simulink library "ITKLib"  (R2022b)
settings: Solver=FixedStepDiscrete  StartTime=0.0  StopTime=10.0  FixedStep=0.01  RelTol=1e-3  EnableMultiTasking=on
values from neighbouring files (symbols this model uses):
  Glb_WhlRollgRd_SC = single(0.36)    [init_Global.m]
undefined symbols (not defined in the file or in its folder): docblock, SlDemoSign, SlDemoSign_Positive_SC, TaskTime_100ms_SC, TaskTime_10ms_SC, VehRefSpd_vMaxRefSpd_C
libraries: simulink x51, $bdroot x45, ITKLib_V14 x1
(part 4 of 10)

== system ITKLib/BasicOperators/AtanDeg ==
  u : Inport
  1-D Lookup Table3 : Lookup_n-D  NumberOfTableDimensions=1  BreakpointsForDimension1=[0,0.00153414561609111,0.00306829845373796,0.00460246573463227,0.00613665468073772,0.00767087251442592,0.00920512645861245,0.0107394237368928,0.0122737715736787,0.0138081771943337,0.0153426478253099,0.0168771906942835,0.0184118130302918,0.0199465220638685,0.0214813250271809,0.0230162291541658,0.0245512416806661,0.0260863698445676,0.0276216208859351,0.0291570020471495,0.0306925205730446,0.0322281837110438,0.0337639987112974,0.0352999728268193,0.0368361133136247,0.0383724274308672,0.0399089224409762,0.0414456056097949,0.0429824842067175,0.0445195655048274,0.0460568567810355,0.0475943653162178,0.0491320983953542,0.0506700633076669,0.0522082673467589,0.0537467178107533,0.0552854220024318,0.0568243872293744,0.0583636208040985,0.0599031300441989,0.0614429222724871,0.0629830048171318,0.0645233850117991,0.0660640701957925,0.0676050677141943,0.0691463849180061,0.0706880291642902,0.0722300078163106,0.0737723282436753,0.0753149978224779,0.0768580239354395,0.0784014139720518,0.0799451753287194,0.0814893154089027,0.0830338416232617,0.0845787613897992,0.0861240821340046,0.0876698112889985,0.089215956295677,0.0907625246028563,0.0923095236674182,0.0938569609544554,0.0954048439374171,0.0969531800982557,0.0985019769275727,0.100051241924766,0.101600982598176,0.103151206465235,0.104701921052615,0.106253133896373,0.107804852542103,0.109357084545084,0.11090983747043,0.112463118893239,0.114016936398742,0.115571297582457,0.117126210050339,0.11868168141893,0.120237719315512,0.12179433137826,0.123351525256394,0.124909308610333,0.126467689111848,0.128026674444216,0.129586272302379,0.131146490393091,0.132707336435082,0.134268818159209,0.135830943308615,0.137393719638886,0.138957154918206,0.140521256927521,0.142086033460691,0.143651492324657,0.145217641339592,0.146784488339068,0.148352041170216,0.149920307693886,0.151489295784808,0.153059013331758,0.15462946823772,0.156200668420048,0.157772621810633,0.159345336356066,0.160918820017808,0.162493080772349,0.164068126611382,0.165643965541967,0.167220605586699,0.168798054783879,0.170376321187682,0.171955412868328,0.173535337912253,0.175116104422279,0.176697720517789,0.178280194334898,0.179863534026628,0.181447747763079,0.183032843731611,0.184618830137013,0.186205715201682,0.187793507165804,0.189382214287526,0.19097184484314,0.192562407127258,0.194153909452998,0.195746360152162,0.197339767575415,0.198934140092477,0.200529486092297,0.202125813983243,0.203723132193287,0.205321449170188,0.206920773381683,0.208521113315675,0.210122477480416,0.211724874404705,0.213328312638072,0.214932800750974,0.216538347334983,0.218144961002985,0.219752650389369,0.221361424150224,0.222971290963538,0.22458225952939,0.226194338570153,0.227807536830688,0.229421863078552,0.231037326104188,0.232653934721138,0.234271697766238,0.235890624099828,0.237510722605954,0.239132002192573,0.240754471791765,0.242378140359935,0.244003016878031,0.245629110351746,0.247256429811733,0.24888498431382,0.250514782939222,0.252145834794754,0.253778149013052,0.255411734752785,0.257046601198878,0.258682757562729,0.260320213082433,0.261958977022998,0.263599058676576,0.265240467362683,0.266883212428424,0.268527303248726,0.270172749226557,0.271819559793166,0.273467744408305,0.275117312560467,0.276768273767119,0.278420637574933,0.280074413560027,0.281729611328199,0.283386240515168,0.285044310786815,0.286703831839422,0.288364813399917,0.290027265226121,0.291691197106988,0.293356618862858,0.295023540345704,0.29669197143938,0.298361922059879,0.300033402155581,0.30170642170751,0.303380990729589,0.305057119268901,0.306734817405947,0.308414095254907,0.310094962963901,0.311777430715259,0.313461508725781,0.315147207247009,0.316834536565492,0.318523507003062,0.320214128917103,0.321906412700828,0.323600368783554,0.325296007630978,0.32699333974546,0.328692375666303,0.330393125970036,0.332095601270698,0.333799812220128,0.33550576950825,0.337213483863366,0.338922966052449,0.340634226881433,0.342347277195516,0.344062127879451,0.345778789857851,0.347497274095491 ...(+13906 chars)]  BreakpointsForDimension1DataTypeStr=single  Table=[0,0.0879,0.1758,0.2637,0.3516,0.4395,0.5274,0.6153,0.7032,0.7911,0.879,0.9669,1.0548,1.1427,1.2306,1.3185,1.4064,1.4943,1.5822,1.6701,1.758,1.8459,1.9338,2.0217,2.1096,2.1975,2.2854,2.3733,2.4612,2.5491,2.637,2.7249,2.8128,2.9007,2.9886,3.0765,3.1644,3.2523,3.3402,3.4281,3.516,3.6039,3.6918,3.7797,3.8676,3.9555,4.0434,4.1313,4.2192,4.3071,4.395,4.4829,4.5708,4.6587,4.7466,4.8345,4.9224,5.0103,5.0982,5.1861,5.274,5.3619,5.4498,5.5377,5.6256,5.7135,5.8014,5.8893,5.9772,6.0651,6.153,6.2409,6.3288,6.4167,6.5046,6.5925,6.6804,6.7683,6.8562,6.9441,7.032,7.1199,7.2078,7.2957,7.3836,7.4715,7.5594,7.6473,7.7352,7.8231,7.911,7.9989,8.0868,8.1747,8.2626,8.3505,8.4384,8.5263,8.6142,8.7021,8.79,8.8779,8.9658,9.0537,9.1416,9.2295,9.3174,9.4053,9.4932,9.5811,9.669,9.7569,9.8448,9.9327,10.0206,10.1085,10.1964,10.2843,10.3722,10.4601,10.548,10.6359,10.7238,10.8117,10.8996,10.9875,11.0754,11.1633,11.2512,11.3391,11.427,11.5149,11.6028,11.6907,11.7786,11.8665,11.9544,12.0423,12.1302,12.2181,12.306,12.3939,12.4818,12.5697,12.6576,12.7455,12.8334,12.9213,13.0092,13.0971,13.185,13.2729,13.3608,13.4487,13.5366,13.6245,13.7124,13.8003,13.8882,13.9761,14.064,14.1519,14.2398,14.3277,14.4156,14.5035,14.5914,14.6793,14.7672,14.8551,14.943,15.0309,15.1188,15.2067,15.2946,15.3825,15.4704,15.5583,15.6462,15.7341,15.822,15.9099,15.9978,16.0857,16.1736,16.2615,16.3494,16.4373,16.5252,16.6131,16.701,16.7889,16.8768,16.9647,17.0526,17.1405,17.2284,17.3163,17.4042,17.4921,17.58,17.6679,17.7558,17.8437,17.9316,18.0195,18.1074,18.1953,18.2832,18.3711,18.459,18.5469,18.6348,18.7227,18.8106,18.8985,18.9864,19.0743,19.1622,19.2501,19.338,19.4259,19.5138,19.6017,19.6896,19.7775,19.8654,19.9533,20.0412,20.1291,20.217,20.3049,20.3928,20.4807,20.5686,20.6565,20.7444,20.8323,20.9202,21.0081,21.096,21.1839,21.2718,21.3597,21.4476,21.5355,21.6234,21.7113,21.7992,21.8871,21.975,22.0629,22.1508,22.2387,22.3266,22.4145,22.5024,22.5903,22.6782,22.7661,22.854,22.9419,23.0298,23.1177,23.2056,23.2935,23.3814,23.4693,23.5572,23.6451,23.733,23.8209,23.9088,23.9967,24.0846,24.1725,24.2604,24.3483,24.4362,24.5241,24.612,24.6999,24.7878,24.8757,24.9636,25.0515,25.1394,25.2273,25.3152,25.4031,25.491,25.5789,25.6668,25.7547,25.8426,25.9305,26.0184,26.1063,26.1942,26.2821,26.37,26.4579,26.5458,26.6337,26.7216,26.8095,26.8974,26.9853,27.0732,27.1611,27.249,27.3369,27.4248,27.5127,27.6006,27.6885,27.7764,27.8643,27.9522,28.0401,28.128,28.2159,28.3038,28.3917,28.4796,28.5675,28.6554,28.7433,28.8312,28.9191,29.007,29.0949,29.1828,29.2707,29.3586,29.4465,29.5344,29.6223,29.7102,29.7981,29.886,29.9739,30.0618,30.1497,30.2376,30.3255,30.4134,30.5013,30.5892,30.6771,30.765,30.8529,30.9408,31.0287,31.1166,31.2045,31.2924,31.3803,31.4682,31.5561,31.644,31.7319,31.8198,31.9077,31.9956,32.0835,32.1714,32.2593,32.3472,32.4351,32.523,32.6109,32.6988,32.7867,32.8746,32.9625,33.0504,33.1383,33.2262,33.3141,33.402,33.4899,33.5778,33.6657,33.7536,33.8415,33.9294,34.0173,34.1052,34.1931,34.281,34.3689,34.4568,34.5447,34.6326,34.7205,34.8084,34.8963,34.9842,35.0721,35.16,35.2479,35.3358,35.4237,35.5116,35.5995,35.6874,35.7753,35.8632,35.9511,36.039,36.1269,36.2148,36.3027,36.3906,36.4785,36.5664,36.6543,36.7422,36.8301,36.918,37.0059,37.0938,37.1817,37.2696,37.3575,37.4454,37.5333,37.6212,37.7091,37.797,37.8849,37.9728,38.0607,38.1486,38.2365,38.3244,38.4123,38.5002,38.5881,38.676,38.7639,38.8518,38.9397,39.0276,39.1155,39.2034,39.2913,39.3792,39.4671,39.555,39.6429,39.7308,39.8187,39.9066,39.9945,40.0824,40.1703,40.2582,40.3461,40.434,40.5219,40.6098,40.6977,40.7856,40.8735,40.9614,41.0493,41.1372,41.2251,41.313,41.4009,41.4888,41.5767,41.6646,41.7525,41.8404,41.9283,42.0162,42.1041,42.192,42.2799,42.3678,42.4557,42.5436,42.6315,42.7194,42.8073,42.8952,42.9831,43.071,43.1589,43.2468,43.3347,43.4226,43.5105,43.5984,43.6863,43.7742,43.8621,43.95,44.0379,44.1258,44.2137,44.3016,44.3895,44.4774,44.5653,44.6532,44.7411,44.829,44.9169,45.0048,45.0927,45.1806,45.2685,45.3564,45.4443,45.5322,45.6201,45.708 ...(+3974 chars)]  TableDataTypeStr=single  IntermediateResultsDataTypeStr=single  ExtrapMethod=Clip  UseLastTableValue=on  InternalRulePriority=Speed  OutDataTypeStr=single  RndMeth=Simplest  FractionDataTypeStr=single
      settings: AttributesFormatString=|
      | input = %<BreakpointsForDimension1>
      | output = %<Table>
      | extrapolation-use end values: %<UseLastTableValue>
  AbsITK : $bdroot/BasicOperators/AbsITK
  GreaterOrEqual3 : RelationalOperator  OutDataTypeStr=boolean
  Product : Product  InputSameDT=on  RndMeth=Zero  SaturateOnIntegerOverflow=on
  Switch1 : Switch  Criteria=u2 ~= 0  SaturateOnIntegerOverflow=off  InputSameDT=off
      settings: AttributesFormatString=Criteria : %<Criteria>
  single1 : Constant  Value=0  OutDataTypeStr=single
      settings: AttributesFormatString=%<OutDataTypeStr>
  single2 : Constant  Value=-1  OutDataTypeStr=single
      settings: AttributesFormatString=%<OutDataTypeStr>
  deg : Outport
  wires:
  single1/1 -> GreaterOrEqual3/2
  GreaterOrEqual3/1 -> Switch1/2
  1-D Lookup Table3/1 -> Product/1, Switch1/1
  Product/1 -> Switch1/3
  Switch1/1 -> deg/1
  u/1 -> AbsITK/1, GreaterOrEqual3/1
  single2/1 -> Product/2
  AbsITK/1 -> 1-D Lookup Table3/1

== system ITKLib/BasicOperators/CosDeg ==
  deg : Inport
  1-D Lookup Table2 : Lookup_n-D  NumberOfTableDimensions=1  BreakpointsForDimension1=[0,5,10,15,20,25,30,35,40,45,50,55,60,65,70,75,80,85,86,87,88,89,90]  BreakpointsForDimension1DataTypeStr=single  Table=[1,0.996194698091746,0.984807753012208,0.965925826289068,0.939692620785908,0.906307787036650,0.866025403784439,0.819152044288992,0.766044443118978,0.707106781186548,0.642787609686539,0.573576436351046,0.500000000000000,0.422618261740699,0.342020143325669,0.258819045102521,0.173648177666930,0.0871557427476584,0.0698,0.0523,0.0349,0.0175,0]  TableDataTypeStr=single  IntermediateResultsDataTypeStr=single  ExtrapMethod=Clip  UseLastTableValue=on  InternalRulePriority=Speed  OutDataTypeStr=single  RndMeth=Simplest  FractionDataTypeStr=single
      settings: AttributesFormatString=|
      | input = %<BreakpointsForDimension1>
      | output = %<Table>
      | extrapolation-use end values: %<UseLastTableValue>
  1-D Lookup Table3 : Lookup_n-D  NumberOfTableDimensions=1  BreakpointsForDimension1=[0,5,10,15,20,25,30,35,40,45,50,55,60,65,70,75,80,85,86,87,88,89,90]  BreakpointsForDimension1DataTypeStr=single  Table=[1,0.996194698091746,0.984807753012208,0.965925826289068,0.939692620785908,0.906307787036650,0.866025403784439,0.819152044288992,0.766044443118978,0.707106781186548,0.642787609686539,0.573576436351046,0.500000000000000,0.422618261740699,0.342020143325669,0.258819045102521,0.173648177666930,0.0871557427476584,0.0698,0.0523,0.0349,0.0175,0]  TableDataTypeStr=single  IntermediateResultsDataTypeStr=single  ExtrapMethod=Clip  UseLastTableValue=on  InternalRulePriority=Speed  OutDataTypeStr=single  RndMeth=Simplest  FractionDataTypeStr=single
      settings: AttributesFormatString=|
      | input = %<BreakpointsForDimension1>
      | output = %<Table>
      | extrapolation-use end values: %<UseLastTableValue>
  AbsITK : $bdroot/BasicOperators/AbsITK
  AbsITK1 : $bdroot/BasicOperators/AbsITK
  Divide : Product  Inputs=*/  InputSameDT=on  RndMeth=Zero  SaturateOnIntegerOverflow=on
  GreaterOrEqual{3..6} (4 alike) : RelationalOperator  OutDataTypeStr=boolean
  GreaterOrEqual7 : RelationalOperator  Operator=<=  OutDataTypeStr=boolean
  GreaterOrEqual8 : RelationalOperator  Operator=<=  OutDataTypeStr=boolean
  GreaterOrEqual9 : RelationalOperator  Operator=<=  OutDataTypeStr=boolean
  Multiport Switch{3..6} (4 alike) : MultiPortSwitch  Inputs=4  SaturateOnIntegerOverflow=off  InputSameDT=off
  Product : Product  InputSameDT=on  RndMeth=Zero  SaturateOnIntegerOverflow=on
  Product2 : Product  InputSameDT=on  RndMeth=Zero  SaturateOnIntegerOverflow=on
  Product3 : Product  InputSameDT=on  RndMeth=Zero  SaturateOnIntegerOverflow=on
  Rounding Function : Rounding  Operator=fix
  Subtract{3..6} (4 alike) : Sum  Inputs=+-  InputSameDT=on  SaturateOnIntegerOverflow=on
  Subtract7 : Sum  InputSameDT=on  SaturateOnIntegerOverflow=on
  Subtract8 : Sum  InputSameDT=on  SaturateOnIntegerOverflow=on
  Switch{1,5..10} (7 alike) : Switch  Criteria=u2 ~= 0  SaturateOnIntegerOverflow=off  InputSameDT=off
      settings: AttributesFormatString=Criteria : %<Criteria>
  single16 : Constant  Value=270  OutDataTypeStr=single
      settings: AttributesFormatString=%<OutDataTypeStr>
  single{4,18,21,30} (4 alike) : Constant  Value=180  OutDataTypeStr=single
      settings: AttributesFormatString=%<OutDataTypeStr>
  single19 : Constant  Value=360  OutDataTypeStr=single
      settings: AttributesFormatString=%<OutDataTypeStr>
  single22 : Constant  Value=360  OutDataTypeStr=single
      settings: AttributesFormatString=%<OutDataTypeStr>
  single23 : Constant  Value=0  OutDataTypeStr=single
      settings: AttributesFormatString=%<OutDataTypeStr>
  single{24,32..33,35} (4 alike) : Constant  OutDataTypeStr=single
      settings: AttributesFormatString=%<OutDataTypeStr>
  single25 : Constant  Value=-1  OutDataTypeStr=single
      settings: AttributesFormatString=%<OutDataTypeStr>
  single27 : Constant  Value=-180  OutDataTypeStr=single
      settings: AttributesFormatString=%<OutDataTypeStr>
  single28 : Constant  Value=-90  OutDataTypeStr=single
      settings: AttributesFormatString=%<OutDataTypeStr>
  single29 : Constant  Value=-270  OutDataTypeStr=single
      settings: AttributesFormatString=%<OutDataTypeStr>
  single3 : Constant  Value=360  OutDataTypeStr=single
      settings: AttributesFormatString=%<OutDataTypeStr>
  single31 : Constant  Value=-1  OutDataTypeStr=single
      settings: AttributesFormatString=%<OutDataTypeStr>
  single8 : Constant  Value=90  OutDataTypeStr=single
      settings: AttributesFormatString=%<OutDataTypeStr>
  uint1 : Constant  OutDataTypeStr=uint8
      settings: AttributesFormatString=%<OutDataTypeStr>
  uint10 : Constant  Value=2  OutDataTypeStr=uint8
      settings: AttributesFormatString=%<OutDataTypeStr>
  uint11 : Constant  Value=3  OutDataTypeStr=uint8
      settings: AttributesFormatString=%<OutDataTypeStr>
  uint12 : Constant  Value=4  OutDataTypeStr=uint8
      settings: AttributesFormatString=%<OutDataTypeStr>
  uint6 : Constant  Value=4  OutDataTypeStr=uint8
      settings: AttributesFormatString=%<OutDataTypeStr>
  uint7 : Constant  Value=3  OutDataTypeStr=uint8
      settings: AttributesFormatString=%<OutDataTypeStr>
  uint8 : Constant  Value=2  OutDataTypeStr=uint8
      settings: AttributesFormatString=%<OutDataTypeStr>
  uint9 : Constant  OutDataTypeStr=uint8
      settings: AttributesFormatString=%<OutDataTypeStr>
  out : Outport
  wires:
  Subtract5/1 -> Multiport Switch3/5
  single23/1 -> GreaterOrEqual6/2
  uint11/1 -> Switch10/1
  single24/1 -> Multiport Switch6/2
  Switch1/1 -> out/1
  GreaterOrEqual4/1 -> Switch6/2
  Product3/1 -> Switch1/3
  Switch8/1 -> Multiport Switch5/1, Multiport Switch6/1
  uint12/1 -> Switch10/3
  GreaterOrEqual5/1 -> Switch7/2
  Subtract4/1 -> Multiport Switch3/4
  GreaterOrEqual6/1 -> Switch1/2
  Switch10/1 -> Switch9/3
  single3/1 -> Product/2, Divide/2
  Switch9/1 -> Switch8/3
  Subtract7/1 -> Multiport Switch5/2
  uint10/1 -> Switch9/1
  1-D Lookup Table2/1 -> Product3/2
  deg/1 -> Divide/1, Subtract6/1
  Divide/1 -> Rounding Function/1
  Product/1 -> Subtract6/2
  Product2/1 -> Switch1/1
  uint6/1 -> Switch5/1
  single16/1 -> GreaterOrEqual3/2
  Switch5/1 -> Multiport Switch3/1, Multiport Switch4/1
  single4/1 -> GreaterOrEqual4/2
  1-D Lookup Table3/1 -> Product2/2
  uint7/1 -> Switch6/1
  Switch6/1 -> Switch5/3
  GreaterOrEqual8/1 -> Switch9/2
  Multiport Switch6/1 -> Product3/1
  uint9/1 -> Switch7/3
  Subtract8/1 -> AbsITK/1, Multiport Switch5/4
  single30/1 -> Subtract3/1
  GreaterOrEqual3/1 -> Switch5/2
  Subtract3/1 -> Multiport Switch3/3
  single28/1 -> GreaterOrEqual9/2
  Rounding Function/1 -> Product/1
  uint1/1 -> Switch8/1
  GreaterOrEqual9/1 -> Switch10/2
  single29/1 -> GreaterOrEqual7/2
  AbsITK/1 -> Multiport Switch5/3
  single25/1 -> Multiport Switch6/3, Multiport Switch6/4
  Multiport Switch3/1 -> 1-D Lookup Table3/1
  Multiport Switch5/1 -> 1-D Lookup Table2/1
  single18/1 -> Subtract4/2
  single19/1 -> Subtract5/1
  GreaterOrEqual7/1 -> Switch8/2
  Multiport Switch4/1 -> Product2/1
  single21/1 -> Subtract8/2
  single27/1 -> GreaterOrEqual8/2
  Switch7/1 -> Switch6/3
  Subtract6/1 -> GreaterOrEqual6/1, AbsITK1/1, Subtract8/1, Subtract7/1, GreaterOrEqual9/1, GreaterOrEqual8/1, GreaterOrEqual7/1, Subtract5/2, Subtract4/1, Subtract3/2, Multiport Switch3/2, GreaterOrEqual5/1, GreaterOrEqual4/1, GreaterOrEqual3/1
  uint8/1 -> Switch7/1
  single8/1 -> GreaterOrEqual5/2
  single22/1 -> Subtract7/2
  single32/1 -> Multiport Switch4/5
  single33/1 -> Multiport Switch4/2
  single31/1 -> Multiport Switch4/3, Multiport Switch4/4
  single35/1 -> Multiport Switch6/5
  AbsITK1/1 -> Multiport Switch5/5

== system ITKLib/BasicOperators/Drvt ==
  In : Inport
  DlyCnt : Inport  Port=2
  dT : Inport  Port=3
  DataTypeConversion : DataTypeConversion  OutDataTypeStr=single  RndMeth=Nearest  SaturateOnIntegerOverflow=off
  Divide1 : Product  Inputs=*/  InputSameDT=on  SaturateOnIntegerOverflow=on
  MaxITK : Subsystem  mask(MaxITK){}
      mask help: This block returns the maximal value of input
      mask Display:
      | color('blue')
      | disp('\fontsize{12}Max', 'texmode', 'on')
      | color('green');
      | text(1,0,'ITK','horizontalAlignment','right','verticalAlignment','bottom');
  Product1 : Product  InputSameDT=on  RndMeth=Zero  SaturateOnIntegerOverflow=on
  Subtract2 : Sum  Inputs=+-  InputSameDT=on  SaturateOnIntegerOverflow=on
  Variable Integer Delay1 : Delay  DelayLengthSource=Input port  DelayLengthUpperLimit=200  UseCircularBuffer=on
      settings: InputPortMap=u0,p1
  Drvt : Outport
  wires:
  DlyCnt/1 -> DataTypeConversion/1, Variable Integer Delay1/2
  Variable Integer Delay1/1 -> Subtract2/2
  MaxITK/1(Out1) -> Divide1/2
  Subtract2/1 -> Divide1/1
  Divide1/1 -> Drvt/1
  In/1 -> Variable Integer Delay1/1, Subtract2/1
  dT/1 -> MaxITK/2(In2), Product1/2
  Product1/1 -> MaxITK/1(In1)
  DataTypeConversion/1 -> Product1/1

== system ITKLib/BasicOperators/Int32ToSingle ==
  In : Inport  OutDataTypeStr=int32
  FL : Inport  Port=2  OutDataTypeStr=single
  DataTypeConversion1 : DataTypeConversion  OutDataTypeStr=single  RndMeth=Nearest
  Divide1 : Product  Inputs=**  SaturateOnIntegerOverflow=on
  Opposite : Subsystem  RTWFcnName=Minus  RTWFileName=MCC_Mdl_Lib  mask(Opposite){}
      mask help:
      | output = - input;
      | Simulink Custom Model Library, created by MCC.
      settings: RTWFcnNameOpts=User specified  RTWFileNameOpts=User specified
      mask Display:
      | color('blue')
      | fprintf('-ln  ')
      | color('green');
      | % text(1,0,'SEN','horizontalAlignment','right','verticalAlignment','bottom');
  Pow : Math  Operator=pow  SignedPower=on  RndMeth=Zero
  single : Constant  Value=2  OutDataTypeStr=single  SampleTime=-1
      settings: AttributesFormatString=%<OutDataTypeStr>
  Out : Outport  OutDataTypeStr=single
  wires:
  DataTypeConversion1/1 -> Out/1
  Opposite/1(" Out ") -> Pow/2
  FL/1 -> Opposite/1(In)
  single/1 -> Pow/1
  Pow/1 -> Divide1/2
  Divide1/1 -> DataTypeConversion1/1
  In/1 -> Divide1/1

== system ITKLib/BasicOperators/MaxITK ==
  In1 : Inport
  In2 : Inport  Port=2
  Greater : RelationalOperator  Operator=>  OutDataTypeStr=boolean
  Switch : Switch  Criteria=u2 ~= 0  SaturateOnIntegerOverflow=off  InputSameDT=off
      settings: AttributesFormatString=Criteria : %<Criteria>
  Out1 : Outport  VectorParamsAs1DForOutWhenUnconnected=off
  wires:
  In1/1 -> Greater/1, Switch/1
  In2/1 -> Switch/3, Greater/2
  Greater/1 -> Switch/2
  Switch/1 -> Out1/1

== system ITKLib/BasicOperators/MinITK ==
  In1 : Inport
  In2 : Inport  Port=2
  Greater : RelationalOperator  Operator=<  OutDataTypeStr=boolean
  Switch : Switch  Criteria=u2 ~= 0  SaturateOnIntegerOverflow=off  InputSameDT=off
      settings: AttributesFormatString=Criteria : %<Criteria>
  Out1 : Outport  VectorParamsAs1DForOutWhenUnconnected=off
  wires:
  Switch/1 -> Out1/1
  Greater/1 -> Switch/2
  In2/1 -> Greater/2, Switch/3
  In1/1 -> Greater/1, Switch/1

== system ITKLib/BasicOperators/ModITK ==
  Dividend : Inport
  Divisor : Inport  Port=2
  Add3 : Sum  Inputs=+-  OutDataTypeStr=Inherit: Inherit via back propagation  RndMeth=Simplest
      settings: AttributesFormatString=|
      | DataType=%<OutDataTypeStr>
      | RndMeth=%<RndMeth>
  Data Type Conversion : DataTypeConversion  OutDataTypeStr=int32  SaturateOnIntegerOverflow=off  RndMeth=Floor
  Divide : Product  Inputs=*/  OutDataTypeStr=Inherit: Inherit via back propagation  RndMeth=Simplest
      settings: AttributesFormatString=RndMeth=%<RndMeth>
  MaxITK : $bdroot/BasicOperators/MaxITK
  Product : Product  Inputs=**  OutDataTypeStr=single  RndMeth=Simplest
      settings: AttributesFormatString=RndMeth=%<RndMeth>
  single : Constant  Value=1e-4  OutDataTypeStr=single  SampleTime=-1
      settings: AttributesFormatString=%<OutDataTypeStr>
  Mod : Outport
  wires:
  Product/1 -> Add3/2
  MaxITK/1 -> Divide/2
  Divide/1 -> Data Type Conversion/1
  single/1 -> MaxITK/1
  Dividend/1 -> Divide/1, Add3/1
  Data Type Conversion/1 -> Product/1
  Add3/1 -> Mod/1
  Divisor/1 -> MaxITK/2, Product/2

== system ITKLib/BasicOperators/Opposite ==
  In : Inport
  Product2 : Product  InputSameDT=on  SaturateOnIntegerOverflow=on
  single : Constant  Value=-1  OutDataTypeStr=single
      settings: AttributesFormatString=%<OutDataTypeStr>
  " Out " : Outport
  wires:
  In/1 -> Product2/1
  Product2/1 -> " Out "/1
  single/1 -> Product2/2

== system ITKLib/BasicOperators/Safe_Divide ==
  In : Inport
  In1 : Inport  Port=2
  eps : Inport  Port=3
  AND : Logic  OutDataTypeStr=boolean
  Abs : Abs  SaturateOnIntegerOverflow=off  OutDataTypeStr=Inherit: Inherit via internal rule
  Divide : Product  Inputs=*/  InputSameDT=on  SaturateOnIntegerOverflow=on
  GreaterOrEqual : RelationalOperator  OutDataTypeStr=boolean
  GreaterOrEqual1 : RelationalOperator  OutDataTypeStr=boolean
  LowerOrEqual : RelationalOperator  Operator=<=  OutDataTypeStr=boolean
  Opposite : Subsystem  RTWFcnName=Minus  RTWFileName=MCC_Mdl_Lib  mask(Opposite){}
      mask help:
      | output = - input;
      | Simulink Custom Model Library, created by MCC.
      settings: RTWFcnNameOpts=User specified  RTWFileNameOpts=User specified
      mask Display:
      | color('blue')
      | fprintf('-ln  ')
      | color('green');
      | % text(1,0,'SEN','horizontalAlignment','right','verticalAlignment','bottom');
  Opposite1 : Subsystem  RTWFcnName=Minus  RTWFileName=MCC_Mdl_Lib  mask(Opposite){}
      mask help:
      | output = - input;
      | Simulink Custom Model Library, created by MCC.
      settings: RTWFcnNameOpts=User specified  RTWFileNameOpts=User specified
      mask Display:
      | color('blue')
      | fprintf('-ln  ')
      | color('green');
      | % text(1,0,'SEN','horizontalAlignment','right','verticalAlignment','bottom');
  Switch : Switch  Criteria=u2 ~= 0  SaturateOnIntegerOverflow=off  InputSameDT=off
      settings: AttributesFormatString=Criteria : %<Criteria>
  Switch1 : Switch  Criteria=u2 ~= 0  SaturateOnIntegerOverflow=off  InputSameDT=off
      settings: AttributesFormatString=Criteria : %<Criteria>
  single : Constant  Value=0  OutDataTypeStr=single
      settings: AttributesFormatString=%<OutDataTypeStr>
  Out : Outport
  wires:
  Switch1/1 -> Switch/1
  [epsAbs] -> Switch1/1
  Opposite1/1(" Out ") -> Switch1/3
  [epsAbs] -> Opposite1/1(In)
  GreaterOrEqual1/1 -> Switch1/2
  [epsAbs] -> Opposite/1(In)
  Opposite/1(" Out ") -> GreaterOrEqual/2
  GreaterOrEqual/1 -> AND/2
  LowerOrEqual/1 -> AND/1
  Abs/1 -> LowerOrEqual/2, [epsAbs]
  eps/1 -> Abs/1
  single/1 -> GreaterOrEqual1/2
  In1/1 -> GreaterOrEqual1/1, LowerOrEqual/1, Switch/3, GreaterOrEqual/1
  AND/1 -> Switch/2
  Switch/1 -> Divide/2
  In/1 -> Divide/1
  Divide/1 -> Out/1
